simulink model "Nernst"  (R2015a)
settings: Solver=ode45  StartTime=0.0  StopTime=100  RelTol=1e-3
libraries: powerlib x4
settings Model: Creator=liu0563  LastModifiedBy=liu0563

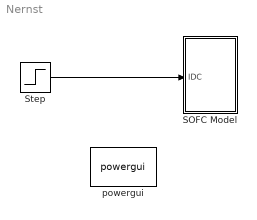
== system Nernst ==
  SOFC Model : Subsystem  mask(Solid Oxide Fuel Cell Model){T=1273, I_FC_0=3.8, F=96.487e6, R=8314, N0=55, U=[0.9 0.8 0.85], K=[8.43e-4 2.81e-4 2.52e-3], taus=[26.1 78.3 2.91], tau_e=0.8, tau_f=5, r_HO=1.145}
      mask prompts: T "Absolute temperature (K)"; I_FC_0 "Initial current (A)"; F "Faraday's constant (C/kmol)"; R "Universal gas constant J/(kmol K)"; N0 "Number of cells in series"; U "Maximum, minimal and optimal fuel utilization"; K "Valve molar constant for hydrogen, water and oxygen (kmol/(s atm)"; taus "Response time for hydrogen, water and oxygen flow (s)"; tau_e "Electrical response time (s)"; tau_f "Fuel processor response time (s)"; r_HO "Ratio of hydrogen to oxygen"
      mask init:
      | U_max=U(1);
      | U_min=U(2);
      | U_opt=U(3);
      | 
      | K_H2=K(1);
      | K_H2O=K(2);
      | K_O2=K(3);
      | 
      | K_r=N0/4/F;
      | 
      | q_H2_0=2*K_r/U_opt*I_FC_0;
      | 
      | p_H2_0=1/K_H2*(q_H2_0-2*K_r*I_FC_0);
      | 
      | p_H2O_0=1/K_H2O*2*K_r*I_FC_0;
      | 
      | p_O2_0=1/K_O2*(1/r_HO*q_H2_0-K_r*I_FC_0);
      | 
      | tau_H2=taus(1);
      | tau_H2O=taus(2);
      | tau_O2=taus(3);
      | 
      | V_Nernst_0=N0*R*T/2/F*log(p_H2_0*sqrt(p_O2_0)/p_H2O_0);
  Step : Step  Time=50  Before=10  After=15  SampleTime=0
  powergui : powerlib/powergui  Priority=1  SimulationMode=Discrete  SolverType=Tustin/Backward Euler (TBE)  SampleTime=0.0005  frequency=60  SPID=off  DisableSnubberDevices=off  DisableRonSwitches=off  DisableVfSwitches=off  SwTol=0  DisplayEquations=off  Interpol=off  methode=off  Ts=100  FunctionMessages=off  echomessages=off  HookPort=off  EnableUseOfTLC=off  x0status=blocks  frequencyindice=0  Pbase=100e6  ErrMax=1e-4  Iterations=50  UnitsV=kV  UnitsW=MW  buscounter=0  RestoreLinks=warning  ResistiveCurrentMeasurement=off  Frange=[0:2:500]  Ylog=off  Xlog=on  ShowGrid=off  save=off  variable=ZData  structure=0  ZoomFFT=off  StartTime=0.0  cycles=1  DisplayStyle=1  fundamental=60  FreqAxis=off  MaxFrequency=1000  frequencyindicesteady=1  RmsSteady=1  display=off
  wires:
  Step/1 -> SOFC Model/1(IDC)

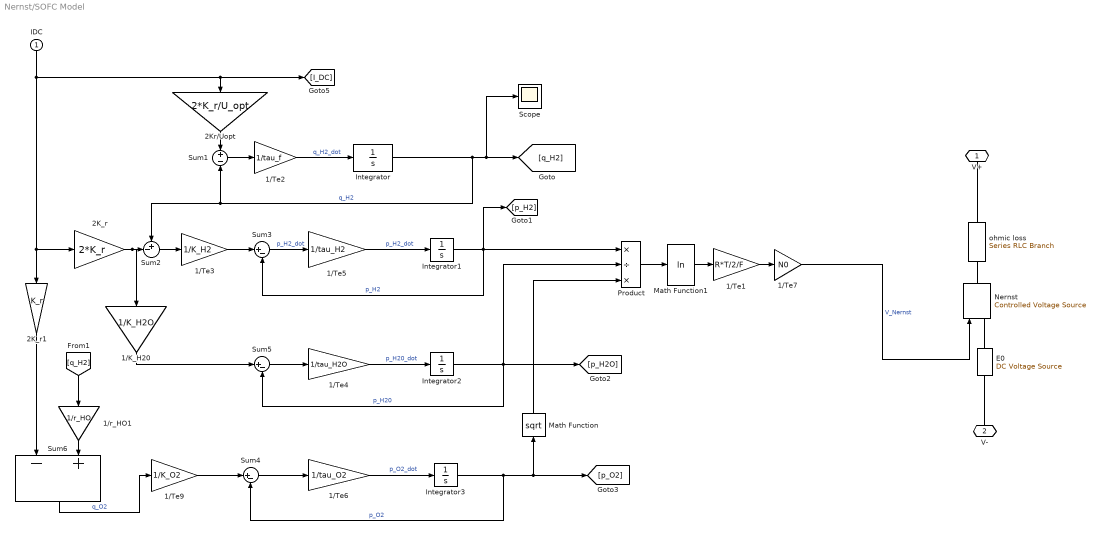
== system Nernst/SOFC Model ==
  IDC : Inport
  1/K_H20 : Gain  Gain=1/K_H2O
  1/Te1 : Gain  Gain=R*T/2/F
  1/Te2 : Gain  Gain=1/tau_f
  1/Te3 : Gain  Gain=1/K_H2
  1/Te4 : Gain  Gain=1/tau_H2O
  1/Te5 : Gain  Gain=1/tau_H2
  1/Te6 : Gain  Gain=1/tau_O2
  1/Te7 : Gain  Gain=N0
  1/Te9 : Gain  Gain=1/K_O2
  1/r_HO1 : Gain  Gain=1/r_HO
  2K_r : Gain  Gain=2*K_r
  2K_r1 : Gain  Gain=K_r
  2Kr/Uopt : Gain  Gain=2*K_r/U_opt
  E0 : powerlib/Electrical Sources/DC Voltage Source  Amplitude=1.18*55  Measurements=None
  Integrator : Integrator  InitialCondition=q_H2_0
  Integrator1 : Integrator  InitialCondition=p_H2_0
  Integrator2 : Integrator  InitialCondition=p_H2O_0
  Integrator3 : Integrator  InitialCondition=p_O2_0
  Math Function : Math  Operator=sqrt  SaturateOnIntegerOverflow=on
  Math Function1 : Math  Operator=log  SaturateOnIntegerOverflow=on
  Nernst : powerlib/Electrical Sources/Controlled Voltage Source  Initialize=on  Source_Type=DC  Amplitude=0  Phase=0  Frequency=0  Measurements=None
  Product : Product  Inputs=*/*  RndMeth=Zero
  Scope : Scope
  Sum1 : Sum  Inputs=+-
  Sum2 : Sum  Inputs=+-|
  Sum3 : Sum  Inputs=|+-
  Sum4 : Sum  Inputs=|+-
  Sum5 : Sum  Inputs=|+-
  Sum6 : Sum  Inputs=-+
  ohmic loss : powerlib/Elements/Series RLC Branch  LConnTagsString=__new0  RConnTagsString=__new0  BranchType=R  Resistance=3.2813e-004*55  Inductance=1.0  SetiL0=off  InitialCurrent=0  Capacitance=1.0  Setx0=off  InitialVoltage=0  Measurements=None
  V+ : PMIOPort  Port=1  Side=Right
  V- : PMIOPort  Port=2  Side=Right
  wires:
  2K_r1/1 -> Sum6/1
  Integrator/1 -> Sum2/1, Sum1/2, Scope/1, [q_H2]  "q_H2"
  Sum6/1 -> 1/Te9/1  "q_O2"
  IDC/1 -> [I_DC], 2Kr/Uopt/1, 2K_r/1, 2K_r1/1
  1/Te7/1 -> Nernst/1  "V_Nernst"
  [q_H2] -> 1/r_HO1/1
  1/Te4/1 -> Integrator2/1  "p_H20_dot"
  Integrator2/1 -> Sum5/2, Product/2, [p_H2O]  "p_H20"
  1/Te2/1 -> Integrator/1  "q_H2_dot"
  Integrator1/1 -> Sum3/2, Product/1, [p_H2]  "p_H2"
  1/r_HO1/1 -> Sum6/2
  Sum3/1 -> 1/Te5/1  "p_H2_dot"
  Sum5/1 -> 1/Te4/1
  1/K_H20/1 -> Sum5/1
  1/Te5/1 -> Integrator1/1  "p_H2_dot"
  Sum4/1 -> 1/Te6/1
  2K_r/1 -> Sum2/2, 1/K_H20/1
  Math Function1/1 -> 1/Te1/1
  1/Te9/1 -> Sum4/1
  1/Te6/1 -> Integrator3/1  "p_O2_dot"
  Integrator3/1 -> Sum4/2, Math Function/1, [p_O2]  "p_O2"
  Sum1/1 -> 1/Te2/1
  2Kr/Uopt/1 -> Sum1/1
  Sum2/1 -> 1/Te3/1
  1/Te3/1 -> Sum3/1
  Math Function/1 -> Product/3
  Product/1 -> Math Function1/1
  1/Te1/1 -> 1/Te7/1
  connections:
  E0/RConn1 -- Nernst/LConn1
  Nernst/RConn1 -- ohmic loss/RConn1
  E0/LConn1 -- V-/RConn1
  V+/RConn1 -- ohmic loss/LConn1
